simulink model "ThreeDOF_cs"  (Simulink 8.8)
settings: Solver=ode5  StartTime=0.0  StopTime=inf  FixedStep=1/20  RelTol=1e-3
model workspace (MAT data in the model file):
  mbox_table : struct (value not decoded)
  model_closed = 0
  sim_status = 0
PreLoadFcn:
  | check_NUTS_defined;
  | 
  | assignin('base',['model_closed_' bdroot],false);
InitFcn:
  | PreScanExperimentInitFcn(bdroot)
StopFcn:
  | PreScanExperimentStopFcn(bdroot)
undefined symbols (not defined in the file): DiscIntNeverNeededParam, InitImageOutputDir
libraries: PreScanSimulinkLibrary x6, PreScanUsefulBlocks x3
(part 1 of 2)
CloseFcn:
  | evalin('base',['clear model_closed_' bdroot]);
settings Model: Creator=PRESCAN  LastModifiedBy=yuntao891011
settings OptimizationCC: ExpressionDepthLimit=2147483647  InitFltsAndDblsToZero=on
settings DebuggingCC: SaveWithParameterizedLinksMsg=none  SignalResolutionControl=TryResolveAllWithWarning  MultiTaskDSMMsg=warning  MultiTaskCondExecSysMsg=none
settings GRTTargetCC: TargetFcnLib=ansi_tfl_tmw.mat

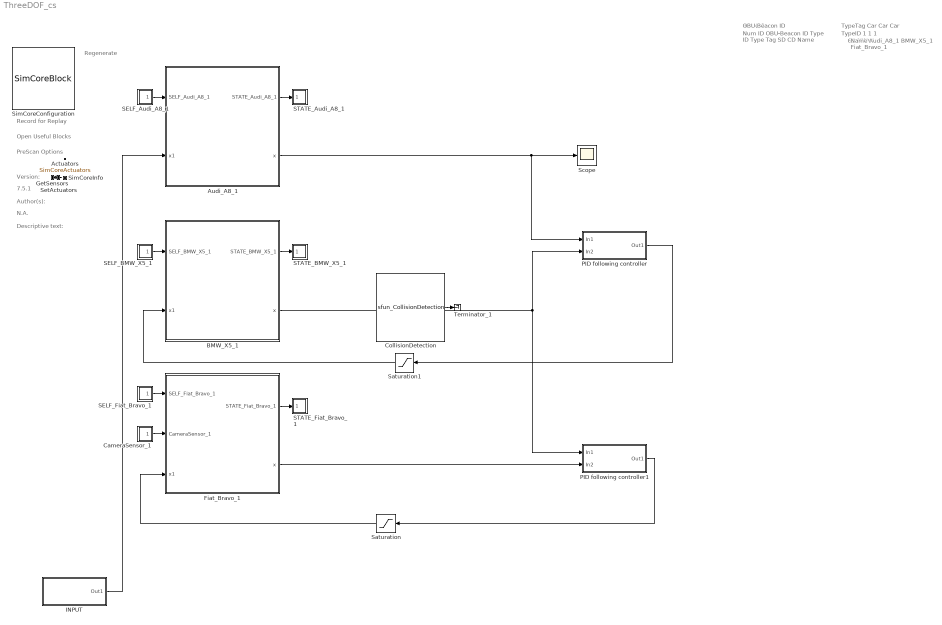
== system ThreeDOF_cs ==
  note: Regenerate
  note: Record for Replay
  note: Open Useful Blocks
  note: PreScan Options
  note: Version:
  note: 7.5.1
  note: Author(s):
  note: N.A.
  note: Descriptive text:
  note: Num ID OBU-Beacon ID Type ID Type Tag SD CD Name
  note: ID
      |
      | 1
      | 2
      | 3
  note: OBU-Beacon ID
  note: TypeID
      |
      | 1
      | 1
      | 1
  note: TypeTag
      |
      | Car
      | Car
      | Car
  note: SD
      |
      | Y
      | Y
      | Y
  note: CD
      |
      | N
      | N
      | N
  note: Name
      |
      | Audi_A8_1
      | BMW_X5_1
      | Fiat_Bravo_1
  Actuators : DataStoreMemory  DataStoreName=SimCoreActuators  InitialValue=zeros(45,1)  ShowAdditionalParam=off
  Audi_A8_1 : Subsystem  Tag=WorldObjectSubSystem  InitFcn=UniqueId = '13';
      mask Display: image(imread('Audi_A8.jpg'));color('white');text(0,0,' ID=1\n')
  BMW_X5_1 : Subsystem  Tag=WorldObjectSubSystem  InitFcn=UniqueId = '14';
      mask Display: image(imread('BMW_X5.jpg'));color('white');text(0,0,' ID=2\n')
  CameraSensor_1 : Subsystem  Tag=CameraSensor  Priority=3  mask(PreScan Source Block: Camera Sensor){}
      mask help: The Camera Sensor provides a color or monochrome image.
      settings: DeleteFcn=PreScanBlockDeleteFcn;
      mask Help: eval('openHelp(457)')
      mask Display: image(imread('CameraSensor.png'))
  CollisionDetection : S-Function  Priority=3  LoadFcn=load('PrescanCollisionDetectionData.mat');load('PrescanCollisionDetectionMessage.mat')  FunctionName=sfun_CollisionDetection  Parameters=timestepMask maxInputMessages maxOutputMessages maxCollisions  SFunctionDeploymentMode=off  EnableBusSupport=off  mask{timestepMask=1/20, maxInputMessages=0, maxOutputMessages=5, maxCollisions=5}
      mask prompts: timestepMask "MATLAB timestep:"; maxInputMessages "Max input messages:"; maxOutputMessages "Max output messages:"; maxCollisions "Maximum number of collisions:"
      mask help: Collision detection output
      mask Display: image(imread('crash.jpg'))
  Fiat_Bravo_1 : Subsystem  Tag=WorldObjectSubSystem  InitFcn=UniqueId = '15';
      mask Display: image(imread('Fiat_Bravo.jpg'));color('white');text(0,0,' ID=3\n')
  GetSensors : Subsystem  Tag=GetSensors  Priority=2  mask(PreScan Simulation Core Block){NrOfSensors=34, TimeStep=1/20}
      mask prompts: NrOfSensors "Number of sensor values"; TimeStep "Timestep [s]"
      mask help:
      | Please do not remove this block from the PreScan compilation sheet,
      | as it contains essential configuration parameters for a PreScan simulation.
      settings: DeleteFcn=PreScanBlockDeleteFcn;
  "INPUT " : Subsystem
  PID following controller : Subsystem
  PID following controller1 : Subsystem
  SELF_Audi_A8_1 : Subsystem  Tag=SELF  Priority=3  mask(PreScan Source Block: SELF){PortName=SELF_Audi_A8_1, PortIndex=10, PortWidth=8, TimeStep=1/20}
      mask prompts: PortName "Auto-Assigned: Port Name [-]"; PortIndex "Auto-Assigned: Port Index [-]"; PortWidth "Auto-Assigned: Port Dimensions"; TimeStep "Auto-Assigned: Upload Period [s]"
      mask help:
      | The SELF port shows (state) information of the actor itself. The outputs are position in the experiment's axis system and the GPS coordinates, and the object's absolute velocity and compass heading.
      |
      | For more information, please click Help.
      settings: DeleteFcn=PreScanBlockDeleteFcn;
      mask Help: eval('openHelp(462)')
      mask Display: image(imread('GPS.png'))
  SELF_BMW_X5_1 : Subsystem  Tag=SELF  Priority=3  mask(PreScan Source Block: SELF){PortName=SELF_BMW_X5_1, PortIndex=18, PortWidth=8, TimeStep=1/20}
      mask prompts: PortName "Auto-Assigned: Port Name [-]"; PortIndex "Auto-Assigned: Port Index [-]"; PortWidth "Auto-Assigned: Port Dimensions"; TimeStep "Auto-Assigned: Upload Period [s]"
      mask help:
      | The SELF port shows (state) information of the actor itself. The outputs are position in the experiment's axis system and the GPS coordinates, and the object's absolute velocity and compass heading.
      |
      | For more information, please click Help.
      settings: DeleteFcn=PreScanBlockDeleteFcn;
      mask Help: eval('openHelp(462)')
      mask Display: image(imread('GPS.png'))
  SELF_Fiat_Bravo_1 : Subsystem  Tag=SELF  Priority=3  mask(PreScan Source Block: SELF){PortName=SELF_Fiat_Bravo_1, PortIndex=26, PortWidth=8, TimeStep=1/20}
      mask prompts: PortName "Auto-Assigned: Port Name [-]"; PortIndex "Auto-Assigned: Port Index [-]"; PortWidth "Auto-Assigned: Port Dimensions"; TimeStep "Auto-Assigned: Upload Period [s]"
      mask help:
      | The SELF port shows (state) information of the actor itself. The outputs are position in the experiment's axis system and the GPS coordinates, and the object's absolute velocity and compass heading.
      |
      | For more information, please click Help.
      settings: DeleteFcn=PreScanBlockDeleteFcn;
      mask Help: eval('openHelp(462)')
      mask Display: image(imread('GPS.png'))
  STATE_Audi_A8_1 : Subsystem  Tag=State  Priority=0  mask(PreScan Sink Block: State){x0=-285.53961181640625, y0=161.16075134277344, z0=0.55, Roll0=0, Pitch0=0, Yaw0=0, TimeStep=1/20}
      mask prompts: x0 "Ini x-position VEHICLE wrt GLOBAL axis system [m]"; y0 "Ini y-position VEHICLE wrt GLOBAL axis system [m]"; z0 "Ini z-position VEHICLE wrt GLOBAL axis system [m]"; Roll0 "Ini roll-angle BODY wrt VEHICLE axis system [deg]"; Pitch0 "Ini pitch-angle BODY wrt VEHICLE axis system [deg]"; Yaw0 "Ini yaw-angle VEHICLE wrt GLOBAL axis system [deg]"; TimeStep "Time Step [s]"
      mask help:
      | The Actor State contains a vector signal of size (9x1), containing the following signals:
      |
      | -  Position                  (x,y,z)                                     [m]
      | -  Velocity                  (vx,vy,vz)                               [m/s]
      | -  Angles                    (Roll, Pitch, Yaw)                   [rad]
      |
      | The Actor state is defined in the global axis system.
      | The state is superponed on the Initial position defined in the GUI.
      |
      | For more information, please click Help.
      settings: DeleteFcn=PreScanBlockDeleteFcn;
      mask Help: eval('openHelp(222)')
      mask Display: image(imread('State.png'))
  STATE_BMW_X5_1 : Subsystem  Tag=State  Priority=0  mask(PreScan Sink Block: State){x0=-302.71296691894531, y0=161.22580718994141, z0=0.69, Roll0=0, Pitch0=0, Yaw0=0, TimeStep=1/20}
      mask prompts: x0 "Ini x-position VEHICLE wrt GLOBAL axis system [m]"; y0 "Ini y-position VEHICLE wrt GLOBAL axis system [m]"; z0 "Ini z-position VEHICLE wrt GLOBAL axis system [m]"; Roll0 "Ini roll-angle BODY wrt VEHICLE axis system [deg]"; Pitch0 "Ini pitch-angle BODY wrt VEHICLE axis system [deg]"; Yaw0 "Ini yaw-angle VEHICLE wrt GLOBAL axis system [deg]"; TimeStep "Time Step [s]"
      mask help:
      | The Actor State contains a vector signal of size (9x1), containing the following signals:
      |
      | -  Position                  (x,y,z)                                     [m]
      | -  Velocity                  (vx,vy,vz)                               [m/s]
      | -  Angles                    (Roll, Pitch, Yaw)                   [rad]
      |
      | The Actor state is defined in the global axis system.
      | The state is superponed on the Initial position defined in the GUI.
      |
      | For more information, please click Help.
      settings: DeleteFcn=PreScanBlockDeleteFcn;
      mask Help: eval('openHelp(222)')
      mask Display: image(imread('State.png'))
  STATE_Fiat_Bravo_1 : Subsystem  Tag=State  Priority=0  mask(PreScan Sink Block: State){x0=-335.43427658081055, y0=161.13351058959961, z0=0.56, Roll0=0, Pitch0=0, Yaw0=0, TimeStep=1/20}
      mask prompts: x0 "Ini x-position VEHICLE wrt GLOBAL axis system [m]"; y0 "Ini y-position VEHICLE wrt GLOBAL axis system [m]"; z0 "Ini z-position VEHICLE wrt GLOBAL axis system [m]"; Roll0 "Ini roll-angle BODY wrt VEHICLE axis system [deg]"; Pitch0 "Ini pitch-angle BODY wrt VEHICLE axis system [deg]"; Yaw0 "Ini yaw-angle VEHICLE wrt GLOBAL axis system [deg]"; TimeStep "Time Step [s]"
      mask help:
      | The Actor State contains a vector signal of size (9x1), containing the following signals:
      |
      | -  Position                  (x,y,z)                                     [m]
      | -  Velocity                  (vx,vy,vz)                               [m/s]
      | -  Angles                    (Roll, Pitch, Yaw)                   [rad]
      |
      | The Actor state is defined in the global axis system.
      | The state is superponed on the Initial position defined in the GUI.
      |
      | For more information, please click Help.
      settings: DeleteFcn=PreScanBlockDeleteFcn;
      mask Help: eval('openHelp(222)')
      mask Display: image(imread('State.png'))
  Saturation : Saturate  UpperLimit=500000  LowerLimit=0
  Saturation1 : Saturate  UpperLimit=500000  LowerLimit=0
  Scope : Scope
  SetActuators : Subsystem  Tag=SetActuators  Priority=1  mask(PreScan Simulation Core Block){TimeStep=1/20, NrOfActuators=45}
      mask prompts: TimeStep "Timestep [s]"; NrOfActuators "Number of actuator values"
      mask help:
      | Please do not remove this block from the PreScan compilation sheet,
      | as it contains essential configuration parameters for a PreScan simulation.
      settings: DeleteFcn=PreScanBlockDeleteFcn;
  SimCoreConfiguration : M-S-Function  Tag=SimCoreConfiguration  Description=DCF5FC37DC6E3E0771C04F3D96D36F9DC5DBC8E5EB9AF2FE837AFFEB0A0E8AE8  FunctionName=SimCoreBlock  Parameters=ExperimentXML PortsXML SimulationCore HostName CheckStart EnableLog RfR EnableGPUAccel ShowComputationTime  mask(PreScan Simulation Core Configurator){SimulationCore=NUTS, HostName=0, CheckStart=0, prescanversion='7.5.1', EnableLog=off, RfR=0, EnableGPUAccel=off, ShowComputationTime=off}
      mask prompts: SimulationCore "Simulation Core"; HostName "Simulation Host"; CheckStart "Show START Dialog"; prescanversion "PreScan Version"; EnableLog "Create TA Log"; RfR "Record for Replay"; EnableGPUAccel "Enable GPU Acceleration"; ShowComputationTime "Show ComputationTime Scope"
      mask help:
      | Please do not remove this block from the PreScan compilation sheet,
      | as it contains essential configuration parameter for a PreScan simulation.
      mask init:
      | model = bdroot;
      | ExperimentXML = [model(1:end-3) '.pex'];
      | PortsXML = [model '_ports.pcd'];
      settings: DeleteFcn=PreScanBlockDeleteFcn;  ModelCloseFcn=assignin('base',['model_closed_' bdroot],true);
      mask Help: eval('openHelp(812)')
      mask Display: image(imread('prescanlogo.ico'))
  SimCoreInfo : Subsystem  Tag=SimCoreInfo
  Terminator_1 : Terminator
  wires:
  SetActuators/1(dummy) -> GetSensors/1(dummy)
  Audi_A8_1/2(x) -> PID following controller/1(In1), Scope/1
  BMW_X5_1/2(x) -> PID following controller1/1(In1), PID following controller/2(In2)
  PID following controller/1(Out1) -> Saturation1/1
  Fiat_Bravo_1/2(x) -> PID following controller1/2(In2)
  PID following controller1/1(Out1) -> Saturation/1
  "INPUT "/1(Out1) -> Audi_A8_1/2(x1)
  Saturation1/1 -> BMW_X5_1/2(x1)
  Saturation/1 -> Fiat_Bravo_1/3(x1)
  Audi_A8_1/1(STATE_Audi_A8_1) -> STATE_Audi_A8_1/1(State)
  SELF_Audi_A8_1/1(U) -> Audi_A8_1/1(SELF_Audi_A8_1)
  BMW_X5_1/1(STATE_BMW_X5_1) -> STATE_BMW_X5_1/1(State)
  SELF_BMW_X5_1/1(U) -> BMW_X5_1/1(SELF_BMW_X5_1)
  Fiat_Bravo_1/1(STATE_Fiat_Bravo_1) -> STATE_Fiat_Bravo_1/1(State)
  SELF_Fiat_Bravo_1/1(U) -> Fiat_Bravo_1/1(SELF_Fiat_Bravo_1)
  CameraSensor_1/1(U1) -> Fiat_Bravo_1/2(CameraSensor_1)
  CollisionDetection/1 -> Terminator_1/1

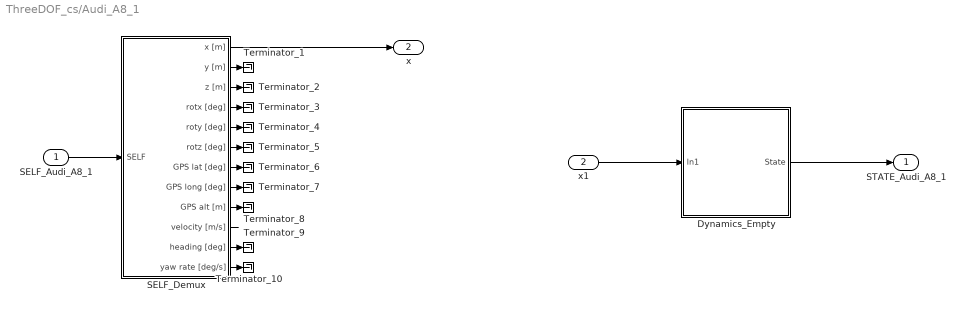
== system ThreeDOF_cs/Audi_A8_1 ==
  SELF_Audi_A8_1 : Inport  Tag=SELFInport
  x1 : Inport  Port=2
  Dynamics_Empty : Subsystem  Tag=Dynamics_Empty
      mask Display: port_label('output', 1, 'State');text(0,0,' Empty\n')
  SELF_Demux : Subsystem  Tag=DemuxSELF  mask(PreScan Demux Block:){}
      settings: DeleteFcn=PreScanBlockDeleteFcn;
      mask Display:
      | port_label('output',1,'x [m]')
      | port_label('output',2,'y [m]')
      | port_label('output',3,'z [m]','texmode','on')
      | port_label('output',4,'Rotx [deg]','texmode','on')
      | port_label('output',5,'Roty [deg]','texmode','on')
      | port_label('output',6,'Rotz [deg]','texmode','on')
      | port_label('output',7,'GPS lat [deg]','texmode','on')
      | port_label('output',8,'GPS long [deg]','texmode','on')
      | port_label('output',9,'GPS alt [m]','texmode','on')
      | port_label('output',10,'Velocity [m/s]')
      | port_label('output',11,'Heading [deg]')
      | port_label('output',12,'Yaw rate [deg/s]')
  Terminator_{1..10} (10 alike) : Terminator
  STATE_Audi_A8_1 : Outport  Tag=StateOutport
  x : Outport  Port=2
  wires:
  SELF_Demux/1(x [m]) -> x/1
  SELF_Demux/10(velocity [m/s]) -> ?
  x1/1 -> Dynamics_Empty/1(In1)
  SELF_Audi_A8_1/1 -> SELF_Demux/1(SELF)
  Dynamics_Empty/1(State) -> STATE_Audi_A8_1/1
  SELF_Demux/2(y [m]) -> Terminator_1/1
  SELF_Demux/3(z [m]) -> Terminator_2/1
  SELF_Demux/4(rotx [deg]) -> Terminator_3/1
  SELF_Demux/5(roty [deg]) -> Terminator_4/1
  SELF_Demux/6(rotz [deg]) -> Terminator_5/1
  SELF_Demux/7(GPS lat [deg]) -> Terminator_6/1
  SELF_Demux/8(GPS long [deg]) -> Terminator_7/1
  SELF_Demux/9(GPS alt [m]) -> Terminator_8/1
  SELF_Demux/11(heading [deg]) -> Terminator_9/1
  SELF_Demux/12(yaw rate [deg/s]) -> Terminator_10/1

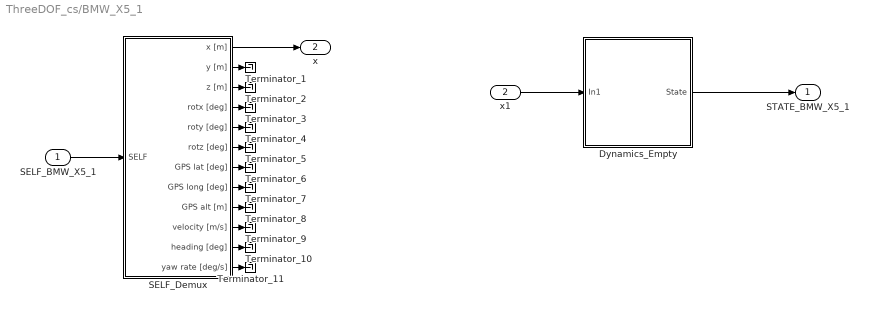
== system ThreeDOF_cs/BMW_X5_1 ==
  SELF_BMW_X5_1 : Inport  Tag=SELFInport
  x1 : Inport  Port=2
  Dynamics_Empty : Subsystem  Tag=Dynamics_Empty
      mask Display: port_label('output', 1, 'State');text(0,0,' Empty\n')
  SELF_Demux : Subsystem  Tag=DemuxSELF  mask(PreScan Demux Block:){}
      settings: DeleteFcn=PreScanBlockDeleteFcn;
      mask Display:
      | port_label('output',1,'x [m]')
      | port_label('output',2,'y [m]')
      | port_label('output',3,'z [m]','texmode','on')
      | port_label('output',4,'Rotx [deg]','texmode','on')
      | port_label('output',5,'Roty [deg]','texmode','on')
      | port_label('output',6,'Rotz [deg]','texmode','on')
      | port_label('output',7,'GPS lat [deg]','texmode','on')
      | port_label('output',8,'GPS long [deg]','texmode','on')
      | port_label('output',9,'GPS alt [m]','texmode','on')
      | port_label('output',10,'Velocity [m/s]')
      | port_label('output',11,'Heading [deg]')
      | port_label('output',12,'Yaw rate [deg/s]')
  Terminator_{1..11} (11 alike) : Terminator
  STATE_BMW_X5_1 : Outport  Tag=StateOutport
  x : Outport  Port=2
  wires:
  SELF_Demux/1(x [m]) -> x/1
  x1/1 -> Dynamics_Empty/1(In1)
  SELF_BMW_X5_1/1 -> SELF_Demux/1(SELF)
  Dynamics_Empty/1(State) -> STATE_BMW_X5_1/1
  SELF_Demux/2(y [m]) -> Terminator_1/1
  SELF_Demux/3(z [m]) -> Terminator_2/1
  SELF_Demux/4(rotx [deg]) -> Terminator_3/1
  SELF_Demux/5(roty [deg]) -> Terminator_4/1
  SELF_Demux/6(rotz [deg]) -> Terminator_5/1
  SELF_Demux/7(GPS lat [deg]) -> Terminator_6/1
  SELF_Demux/8(GPS long [deg]) -> Terminator_7/1
  SELF_Demux/9(GPS alt [m]) -> Terminator_8/1
  SELF_Demux/10(velocity [m/s]) -> Terminator_9/1
  SELF_Demux/11(heading [deg]) -> Terminator_10/1
  SELF_Demux/12(yaw rate [deg/s]) -> Terminator_11/1

== system ThreeDOF_cs/CameraSensor_1 ==
  Demux : Demux  Outputs=[1 -1]
  Terminator : Terminator
  U1 : Outport
  wires:
  Demux/2 -> Terminator/1
  Demux/1 -> U1/1
  [SimCoreSensors] -> Demux/1

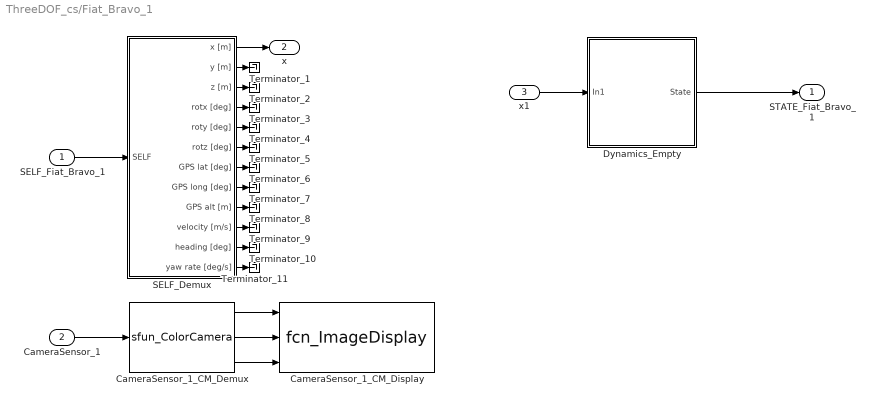
== system ThreeDOF_cs/Fiat_Bravo_1 ==
  SELF_Fiat_Bravo_1 : Inport  Tag=SELFInport
  CameraSensor_1 : Inport  Tag=CameraSensorInport  Port=2  SampleTime=1/20
  x1 : Inport  Port=3
  CameraSensor_1_CM_Demux : S-Function  Tag=CameraSensor_Color_Demux  FunctionName=sfun_ColorCamera  Parameters=[VerticalResolution HorizontalResolution] FrameRate SensorName CameraType SharedMemTag SharedMemRightTag DataType  SFunctionDeploymentMode=off  EnableBusSupport=off  mask{HorizontalResolution=500, VerticalResolution=375, FrameRate=20, SensorName=CameraSensor_1, CameraType=Mono, SharedMemTag=CameraSensor_1_monoBeam_viewer_RGB, SharedMemRightTag=CameraSensor_1_StereoRight_viewer_RGB, DataType=uint8}
      mask prompts: HorizontalResolution "User Specified: Horizontal Resolution [pixels]"; VerticalResolution "User Specified: Vertical Resolution [pixels]"; FrameRate "User Specified: Frame Rate [Hz]"; SensorName "User Specified: Camera Sensor Name"; CameraType "Camera Type"; SharedMemTag "Tag for shared memory for main img"; SharedMemRightTag "Tag for shared memory for right img"; DataType "Image Data Type"
      mask init:
      | if CameraType==1
      |     CameraTypeName='MONO';
      |     PortNumber=0;
      | else
      |     CameraTypeName='STEREO';
      |     PortNumber=3;
      | end
      settings: DeleteFcn=PreScanBlockDeleteFcn;
      mask TypeOptions CameraType: Mono | Stereo
      mask TypeOptions DataType: uint8 | single
      mask Display:
      | fprintf('%s CAMERA:\n Color\n %s \n V: %d x %d \n %d fps',CameraTypeName,SensorName,VerticalResolution,HorizontalResolution,FrameRate)
      | port_label('output',1,'R')
      | port_label('output',2,'G')
      | port_label('output',3,'B')
      | port_label('output',PortNumber+1,'R')
      | port_label('output',PortNumber+2,'G')
      | port_label('output',PortNumber+3,'B')
  CameraSensor_1_CM_Display : M-S-Function  Tag=CameraSensor_Color_Display  InitFcn=InitImageOutputDir(gcb);  FunctionName=fcn_ImageDisplay  Parameters=SensorName EnableDisplay EnablePosition DisplayPosition FigureHandle SaveResults BitmapFormat TempOutputDir CameraType DataType  mask(PreScan Color Display Block){SensorName=CameraSensor_1, EnableDisplay=on, EnablePosition=off, DisplayPosition=[10 10 500 375], FigureHandle=300, SaveResults=off, Format=PNG, TempOutputDir=0, CameraType=Mono, DataType=uint8}
      mask prompts: SensorName "User Specified: Title of Display"; EnableDisplay "Active"; EnablePosition "Set Display window position"; DisplayPosition "Display window position [xpos ypos width height]"; FigureHandle "Unique Handle"; SaveResults "Save results"; TempOutputDir "OutputDir"; CameraType "Camera Type"; DataType "Image Data Type"
      mask help: This block displays the RGB output of a PreScan camera sensor.
      mask init:
      | if EnableDisplay
      |     EnableString='';
      |     EnableColor='gray';
      | else
      |     EnableString='INACTIVE';
      |     EnableColor='red';
      | end
      | switch Format
      |     case 1
      |         BitmapFormat = 'png';
      |     case 2
      |         BitmapFormat = 'bmp';
      |     case 3
      |         BitmapFormat = 'jpg';
      | end 
      | if CameraType==1
      |     CameraTypeName='MONO';
      |     PortNumber=0;
      | else
      |     CameraTypeName='STEREO';
      |     PortNumber=3;
      | end
      settings: CopyFcn=CopyFcnDisplay  DeleteFcn=PreScanBlockDeleteFcn;  ModelCloseFcn=fcn_ImageDisplay_ModelCloseFcn
      mask Help: eval('openHelp(457)')
      mask Callback EnablePosition:
      | MV=get_param(gcb,'MaskVisibilities');
      | if strcmp(get_param(gcb,'EnablePosition'),'on')
      |     MV{4}='on';
      | else
      |     MV{4}='off';
      | end
      | set_param(gcb,'MaskVisibilities',MV);
      mask TypeOptions Format: PNG | BMP | JPG
      mask TypeOptions CameraType: Mono | Stereo
      mask TypeOptions DataType: uint8 | single
      mask Display:
      | color(EnableColor);
      | fprintf('%s\n DISPLAY:\n Color \n %s',EnableString,SensorName)
      | port_label('input',1,'R')
      | port_label('input',2,'G')
      | port_label('input',3,'B')
      | port_label('input',PortNumber+1,'R')
      | port_label('input',PortNumber+2,'G')
      | port_label('input',PortNumber+3,'B')
  Dynamics_Empty : Subsystem  Tag=Dynamics_Empty
      mask Display: port_label('output', 1, 'State');text(0,0,' Empty\n')
  SELF_Demux : Subsystem  Tag=DemuxSELF  mask(PreScan Demux Block:){}
      settings: DeleteFcn=PreScanBlockDeleteFcn;
      mask Display:
      | port_label('output',1,'x [m]')
      | port_label('output',2,'y [m]')
      | port_label('output',3,'z [m]','texmode','on')
      | port_label('output',4,'Rotx [deg]','texmode','on')
      | port_label('output',5,'Roty [deg]','texmode','on')
      | port_label('output',6,'Rotz [deg]','texmode','on')
      | port_label('output',7,'GPS lat [deg]','texmode','on')
      | port_label('output',8,'GPS long [deg]','texmode','on')
      | port_label('output',9,'GPS alt [m]','texmode','on')
      | port_label('output',10,'Velocity [m/s]')
      | port_label('output',11,'Heading [deg]')
      | port_label('output',12,'Yaw rate [deg/s]')
  Terminator_{1..11} (11 alike) : Terminator
  STATE_Fiat_Bravo_1 : Outport  Tag=StateOutport
  x : Outport  Port=2
  wires:
  SELF_Demux/1(x [m]) -> x/1
  x1/1 -> Dynamics_Empty/1(In1)
  SELF_Fiat_Bravo_1/1 -> SELF_Demux/1(SELF)
  CameraSensor_1_CM_Demux/1 -> CameraSensor_1_CM_Display/1
  CameraSensor_1_CM_Demux/2 -> CameraSensor_1_CM_Display/2
  CameraSensor_1_CM_Demux/3 -> CameraSensor_1_CM_Display/3
  CameraSensor_1/1 -> CameraSensor_1_CM_Demux/1
  Dynamics_Empty/1(State) -> STATE_Fiat_Bravo_1/1
  SELF_Demux/2(y [m]) -> Terminator_1/1
  SELF_Demux/3(z [m]) -> Terminator_2/1
  SELF_Demux/4(rotx [deg]) -> Terminator_3/1
  SELF_Demux/5(roty [deg]) -> Terminator_4/1
  SELF_Demux/6(rotz [deg]) -> Terminator_5/1
  SELF_Demux/7(GPS lat [deg]) -> Terminator_6/1
  SELF_Demux/8(GPS long [deg]) -> Terminator_7/1
  SELF_Demux/9(GPS alt [m]) -> Terminator_8/1
  SELF_Demux/10(velocity [m/s]) -> Terminator_9/1
  SELF_Demux/11(heading [deg]) -> Terminator_10/1
  SELF_Demux/12(yaw rate [deg/s]) -> Terminator_11/1

== system ThreeDOF_cs/GetSensors ==
  dummy : Inport
  GetSensors : M-S-Function  FunctionName=GetSensorsBlock  Parameters=TimeStep NrOfSensors
  tag scope: SimCoreSensors=global
  wires:
  GetSensors/1 -> [SimCoreSensors]
  dummy/1 -> GetSensors/1

== system ThreeDOF_cs/INPUT  ==
  Scope : Scope
  Sine Wave : Sin  Amplitude=2  Bias=2.5  Frequency=0.4  SampleTime=0
  Out1 : Outport
  wires:
  Sine Wave/1 -> Scope/1, Out1/1

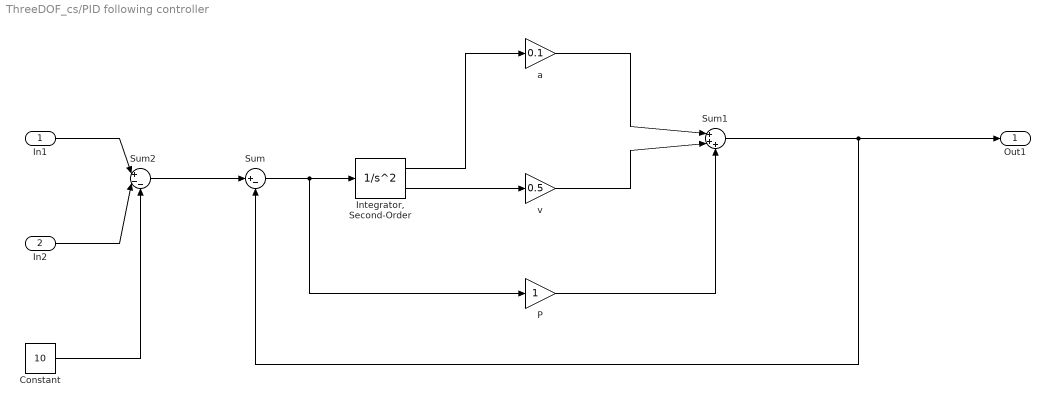
== system ThreeDOF_cs/PID following controller ==
  In1 : Inport
  In2 : Inport  Port=2
  Constant : Constant  Value=10
  "Integrator, Second-Order" : SecondOrderIntegrator
  P : Gain
  Sum : Sum  Inputs=|+-
  Sum1 : Sum  Inputs=|+++
  Sum2 : Sum  Inputs=|+--
  a : Gain  Gain=0.1
  v : Gain  Gain=0.5
  Out1 : Outport
  wires:
  Sum/1 -> P/1, "Integrator, Second-Order"/1
  "Integrator, Second-Order"/1 -> a/1
  "Integrator, Second-Order"/2 -> v/1
  a/1 -> Sum1/1
  v/1 -> Sum1/2
  P/1 -> Sum1/3
  Sum1/1 -> Out1/1, Sum/2
  In1/1 -> Sum2/1
  Sum2/1 -> Sum/1
  In2/1 -> Sum2/2
  Constant/1 -> Sum2/3

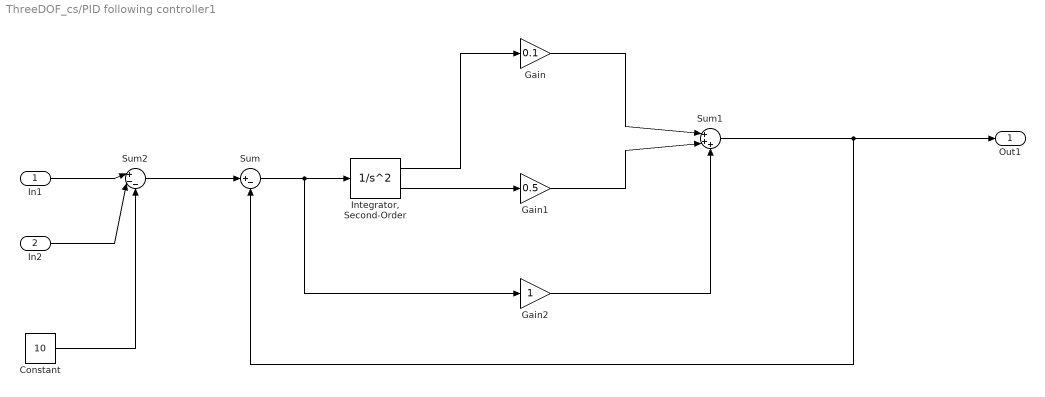
== system ThreeDOF_cs/PID following controller1 ==
  In1 : Inport
  In2 : Inport  Port=2
  Constant : Constant  Value=10
  Gain : Gain  Gain=0.1
  Gain1 : Gain  Gain=0.5
  Gain2 : Gain
  "Integrator, Second-Order" : SecondOrderIntegrator
  Sum : Sum  Inputs=|+-
  Sum1 : Sum  Inputs=|+++
  Sum2 : Sum  Inputs=|+--
  Out1 : Outport
  wires:
  Sum/1 -> Gain2/1, "Integrator, Second-Order"/1
  "Integrator, Second-Order"/1 -> Gain/1
  "Integrator, Second-Order"/2 -> Gain1/1
  Gain/1 -> Sum1/1
  Gain1/1 -> Sum1/2
  Gain2/1 -> Sum1/3
  Sum1/1 -> Out1/1, Sum/2
  In1/1 -> Sum2/1
  Sum2/1 -> Sum/1
  In2/1 -> Sum2/2
  Constant/1 -> Sum2/3

== system ThreeDOF_cs/SELF_Audi_A8_1 ==
  Selector : Selector  IndexMode=Zero-based  IndexOptions=Starting index (dialog)  Indices=PortIndex  OutputSizes=PortWidth(1)
  U : Outport
  wires:
  Selector/1 -> U/1
  [SimCoreSensors] -> Selector/1

== system ThreeDOF_cs/SELF_BMW_X5_1 ==
  Selector : Selector  IndexMode=Zero-based  IndexOptions=Starting index (dialog)  Indices=PortIndex  OutputSizes=PortWidth(1)
  U : Outport
  wires:
  Selector/1 -> U/1
  [SimCoreSensors] -> Selector/1

== system ThreeDOF_cs/SELF_Fiat_Bravo_1 ==
  Selector : Selector  IndexMode=Zero-based  IndexOptions=Starting index (dialog)  Indices=PortIndex  OutputSizes=PortWidth(1)
  U : Outport
  wires:
  Selector/1 -> U/1
  [SimCoreSensors] -> Selector/1

== system ThreeDOF_cs/STATE_Audi_A8_1 ==
  State : Inport  SampleTime=TimeStep
  Acceleration : Subsystem  mask(ToSensorWorld){PortName=Acceleration_Audi_A8_1, PortIndex=6, PortWidth=3, TimeStep=1/20}
      mask prompts: PortName "Port Name [-]"; PortIndex "Index [-]"; PortWidth "Port Dimensions [-]"; TimeStep "Upload Period [s]"
      mask help: Sends signal(s) from Simulink to the Sensor World
      mask Help:
      | Sends signal(s) from Simulink to the Sensor World.
      | 
      | - Port Name [-]: specifies the name of the output terminal of the Simulink block.
      | - Index [-]: specifies the start position in the output vector sent to the Sensor World
      | - Port dimensions [-]: specifies the width (number of scalars) of the output port
      | - Upload period [s]: specifies the upload period (in seconds) of the port.
      mask Display: port_label('input', 1, PortName)
  Demux : Demux  Outputs=5
  Position : Subsystem  mask(ToSensorWorld){PortName=Position_Audi_A8_1, PortIndex=0, PortWidth=3, TimeStep=1/20}
      mask prompts: PortName "Port Name [-]"; PortIndex "Index [-]"; PortWidth "Port Dimensions [-]"; TimeStep "Upload Period [s]"
      mask help: Sends signal(s) from Simulink to the Sensor World
      mask Help:
      | Sends signal(s) from Simulink to the Sensor World.
      | 
      | - Port Name [-]: specifies the name of the output terminal of the Simulink block.
      | - Index [-]: specifies the start position in the output vector sent to the Sensor World
      | - Port dimensions [-]: specifies the width (number of scalars) of the output port
      | - Upload period [s]: specifies the upload period (in seconds) of the port.
      mask Display: port_label('input', 1, PortName)
  RPY : Subsystem  mask(ToSensorWorld){PortName=RPY_Audi_A8_1, PortIndex=9, PortWidth=3, TimeStep=1/20}
      mask prompts: PortName "Port Name [-]"; PortIndex "Index [-]"; PortWidth "Port Dimensions [-]"; TimeStep "Upload Period [s]"
      mask help: Sends signal(s) from Simulink to the Sensor World
      mask Help:
      | Sends signal(s) from Simulink to the Sensor World.
      | 
      | - Port Name [-]: specifies the name of the output terminal of the Simulink block.
      | - Index [-]: specifies the start position in the output vector sent to the Sensor World
      | - Port dimensions [-]: specifies the width (number of scalars) of the output port
      | - Upload period [s]: specifies the upload period (in seconds) of the port.
      mask Display: port_label('input', 1, PortName)
  Velocity : Subsystem  mask(ToSensorWorld){PortName=Velocity_Audi_A8_1, PortIndex=3, PortWidth=3, TimeStep=1/20}
      mask prompts: PortName "Port Name [-]"; PortIndex "Index [-]"; PortWidth "Port Dimensions [-]"; TimeStep "Upload Period [s]"
      mask help: Sends signal(s) from Simulink to the Sensor World
      mask Help:
      | Sends signal(s) from Simulink to the Sensor World.
      | 
      | - Port Name [-]: specifies the name of the output terminal of the Simulink block.
      | - Index [-]: specifies the start position in the output vector sent to the Sensor World
      | - Port dimensions [-]: specifies the width (number of scalars) of the output port
      | - Upload period [s]: specifies the upload period (in seconds) of the port.
      mask Display: port_label('input', 1, PortName)
  iniBODYAngles wrtVEH [rad] : Constant  Value=[Roll0 Pitch0 0]  SampleTime=TimeStep
  iniVEHAngles wrtGLOB [rad] : Constant  Value=[0 0 Yaw0]  SampleTime=TimeStep
  iniVEHposition wrtGLOB [m] : Constant  Value=[x0 y0 z0]  SampleTime=TimeStep
  state2FullState : PreScanSimulinkLibrary/state2FullState  SystemSampleTime=-1
  velRPY : Subsystem  mask(ToSensorWorld){PortName=velRPY_Audi_A8_1, PortIndex=12, PortWidth=3, TimeStep=1/20}
      mask prompts: PortName "Port Name [-]"; PortIndex "Index [-]"; PortWidth "Port Dimensions [-]"; TimeStep "Upload Period [s]"
      mask help: Sends signal(s) from Simulink to the Sensor World
      mask Help:
      | Sends signal(s) from Simulink to the Sensor World.
      | 
      | - Port Name [-]: specifies the name of the output terminal of the Simulink block.
      | - Index [-]: specifies the start position in the output vector sent to the Sensor World
      | - Port dimensions [-]: specifies the width (number of scalars) of the output port
      | - Upload period [s]: specifies the upload period (in seconds) of the port.
      mask Display: port_label('input', 1, PortName)
  wires:
  Demux/5 -> velRPY/1(Y)
  Demux/4 -> RPY/1(Y)
  Demux/3 -> Acceleration/1(Y)
  Demux/2 -> Velocity/1(Y)
  Demux/1 -> Position/1(Y)
  State/1 -> state2FullState/1
  state2FullState/1 -> Demux/1
  iniVEHposition wrtGLOB [m]/1 -> state2FullState/2
  iniBODYAngles wrtVEH [rad]/1 -> state2FullState/3
  iniVEHAngles wrtGLOB [rad]/1 -> state2FullState/4

== system ThreeDOF_cs/STATE_BMW_X5_1 ==
  State : Inport  SampleTime=TimeStep
  Acceleration : Subsystem  mask(ToSensorWorld){PortName=Acceleration_BMW_X5_1, PortIndex=21, PortWidth=3, TimeStep=1/20}
      mask prompts: PortName "Port Name [-]"; PortIndex "Index [-]"; PortWidth "Port Dimensions [-]"; TimeStep "Upload Period [s]"
      mask help: Sends signal(s) from Simulink to the Sensor World
      mask Help:
      | Sends signal(s) from Simulink to the Sensor World.
      | 
      | - Port Name [-]: specifies the name of the output terminal of the Simulink block.
      | - Index [-]: specifies the start position in the output vector sent to the Sensor World
      | - Port dimensions [-]: specifies the width (number of scalars) of the output port
      | - Upload period [s]: specifies the upload period (in seconds) of the port.
      mask Display: port_label('input', 1, PortName)
  Demux : Demux  Outputs=5
  Position : Subsystem  mask(ToSensorWorld){PortName=Position_BMW_X5_1, PortIndex=15, PortWidth=3, TimeStep=1/20}
      mask prompts: PortName "Port Name [-]"; PortIndex "Index [-]"; PortWidth "Port Dimensions [-]"; TimeStep "Upload Period [s]"
      mask help: Sends signal(s) from Simulink to the Sensor World
      mask Help:
      | Sends signal(s) from Simulink to the Sensor World.
      | 
      | - Port Name [-]: specifies the name of the output terminal of the Simulink block.
      | - Index [-]: specifies the start position in the output vector sent to the Sensor World
      | - Port dimensions [-]: specifies the width (number of scalars) of the output port
      | - Upload period [s]: specifies the upload period (in seconds) of the port.
      mask Display: port_label('input', 1, PortName)
  RPY : Subsystem  mask(ToSensorWorld){PortName=RPY_BMW_X5_1, PortIndex=24, PortWidth=3, TimeStep=1/20}
      mask prompts: PortName "Port Name [-]"; PortIndex "Index [-]"; PortWidth "Port Dimensions [-]"; TimeStep "Upload Period [s]"
      mask help: Sends signal(s) from Simulink to the Sensor World
      mask Help:
      | Sends signal(s) from Simulink to the Sensor World.
      | 
      | - Port Name [-]: specifies the name of the output terminal of the Simulink block.
      | - Index [-]: specifies the start position in the output vector sent to the Sensor World
      | - Port dimensions [-]: specifies the width (number of scalars) of the output port
      | - Upload period [s]: specifies the upload period (in seconds) of the port.
      mask Display: port_label('input', 1, PortName)
  Velocity : Subsystem  mask(ToSensorWorld){PortName=Velocity_BMW_X5_1, PortIndex=18, PortWidth=3, TimeStep=1/20}
      mask prompts: PortName "Port Name [-]"; PortIndex "Index [-]"; PortWidth "Port Dimensions [-]"; TimeStep "Upload Period [s]"
      mask help: Sends signal(s) from Simulink to the Sensor World
      mask Help:
      | Sends signal(s) from Simulink to the Sensor World.
      | 
      | - Port Name [-]: specifies the name of the output terminal of the Simulink block.
      | - Index [-]: specifies the start position in the output vector sent to the Sensor World
      | - Port dimensions [-]: specifies the width (number of scalars) of the output port
      | - Upload period [s]: specifies the upload period (in seconds) of the port.
      mask Display: port_label('input', 1, PortName)
  iniBODYAngles wrtVEH [rad] : Constant  Value=[Roll0 Pitch0 0]  SampleTime=TimeStep
  iniVEHAngles wrtGLOB [rad] : Constant  Value=[0 0 Yaw0]  SampleTime=TimeStep
  iniVEHposition wrtGLOB [m] : Constant  Value=[x0 y0 z0]  SampleTime=TimeStep
  state2FullState : PreScanSimulinkLibrary/state2FullState  SystemSampleTime=-1
  velRPY : Subsystem  mask(ToSensorWorld){PortName=velRPY_BMW_X5_1, PortIndex=27, PortWidth=3, TimeStep=1/20}
      mask prompts: PortName "Port Name [-]"; PortIndex "Index [-]"; PortWidth "Port Dimensions [-]"; TimeStep "Upload Period [s]"
      mask help: Sends signal(s) from Simulink to the Sensor World
      mask Help:
      | Sends signal(s) from Simulink to the Sensor World.
      | 
      | - Port Name [-]: specifies the name of the output terminal of the Simulink block.
      | - Index [-]: specifies the start position in the output vector sent to the Sensor World
      | - Port dimensions [-]: specifies the width (number of scalars) of the output port
      | - Upload period [s]: specifies the upload period (in seconds) of the port.
      mask Display: port_label('input', 1, PortName)
  wires:
  Demux/5 -> velRPY/1(Y)
  Demux/4 -> RPY/1(Y)
  Demux/3 -> Acceleration/1(Y)
  Demux/2 -> Velocity/1(Y)
  Demux/1 -> Position/1(Y)
  State/1 -> state2FullState/1
  state2FullState/1 -> Demux/1
  iniVEHposition wrtGLOB [m]/1 -> state2FullState/2
  iniBODYAngles wrtVEH [rad]/1 -> state2FullState/3
  iniVEHAngles wrtGLOB [rad]/1 -> state2FullState/4

== system ThreeDOF_cs/STATE_Fiat_Bravo_1 ==
  State : Inport  SampleTime=TimeStep
  Acceleration : Subsystem  mask(ToSensorWorld){PortName=Acceleration_Fiat_Bravo_1, PortIndex=36, PortWidth=3, TimeStep=1/20}
      mask prompts: PortName "Port Name [-]"; PortIndex "Index [-]"; PortWidth "Port Dimensions [-]"; TimeStep "Upload Period [s]"
      mask help: Sends signal(s) from Simulink to the Sensor World
      mask Help:
      | Sends signal(s) from Simulink to the Sensor World.
      | 
      | - Port Name [-]: specifies the name of the output terminal of the Simulink block.
      | - Index [-]: specifies the start position in the output vector sent to the Sensor World
      | - Port dimensions [-]: specifies the width (number of scalars) of the output port
      | - Upload period [s]: specifies the upload period (in seconds) of the port.
      mask Display: port_label('input', 1, PortName)
  Demux : Demux  Outputs=5
  Position : Subsystem  mask(ToSensorWorld){PortName=Position_Fiat_Bravo_1, PortIndex=30, PortWidth=3, TimeStep=1/20}
      mask prompts: PortName "Port Name [-]"; PortIndex "Index [-]"; PortWidth "Port Dimensions [-]"; TimeStep "Upload Period [s]"
      mask help: Sends signal(s) from Simulink to the Sensor World
      mask Help:
      | Sends signal(s) from Simulink to the Sensor World.
      | 
      | - Port Name [-]: specifies the name of the output terminal of the Simulink block.
      | - Index [-]: specifies the start position in the output vector sent to the Sensor World
      | - Port dimensions [-]: specifies the width (number of scalars) of the output port
      | - Upload period [s]: specifies the upload period (in seconds) of the port.
      mask Display: port_label('input', 1, PortName)
  RPY : Subsystem  mask(ToSensorWorld){PortName=RPY_Fiat_Bravo_1, PortIndex=39, PortWidth=3, TimeStep=1/20}
      mask prompts: PortName "Port Name [-]"; PortIndex "Index [-]"; PortWidth "Port Dimensions [-]"; TimeStep "Upload Period [s]"
      mask help: Sends signal(s) from Simulink to the Sensor World
      mask Help:
      | Sends signal(s) from Simulink to the Sensor World.
      | 
      | - Port Name [-]: specifies the name of the output terminal of the Simulink block.
      | - Index [-]: specifies the start position in the output vector sent to the Sensor World
      | - Port dimensions [-]: specifies the width (number of scalars) of the output port
      | - Upload period [s]: specifies the upload period (in seconds) of the port.
      mask Display: port_label('input', 1, PortName)
  Velocity : Subsystem  mask(ToSensorWorld){PortName=Velocity_Fiat_Bravo_1, PortIndex=33, PortWidth=3, TimeStep=1/20}
      mask prompts: PortName "Port Name [-]"; PortIndex "Index [-]"; PortWidth "Port Dimensions [-]"; TimeStep "Upload Period [s]"
      mask help: Sends signal(s) from Simulink to the Sensor World
      mask Help:
      | Sends signal(s) from Simulink to the Sensor World.
      | 
      | - Port Name [-]: specifies the name of the output terminal of the Simulink block.
      | - Index [-]: specifies the start position in the output vector sent to the Sensor World
      | - Port dimensions [-]: specifies the width (number of scalars) of the output port
      | - Upload period [s]: specifies the upload period (in seconds) of the port.
      mask Display: port_label('input', 1, PortName)
  iniBODYAngles wrtVEH [rad] : Constant  Value=[Roll0 Pitch0 0]  SampleTime=TimeStep
  iniVEHAngles wrtGLOB [rad] : Constant  Value=[0 0 Yaw0]  SampleTime=TimeStep
  iniVEHposition wrtGLOB [m] : Constant  Value=[x0 y0 z0]  SampleTime=TimeStep
  state2FullState : PreScanSimulinkLibrary/state2FullState  SystemSampleTime=-1
  velRPY : Subsystem  mask(ToSensorWorld){PortName=velRPY_Fiat_Bravo_1, PortIndex=42, PortWidth=3, TimeStep=1/20}
      mask prompts: PortName "Port Name [-]"; PortIndex "Index [-]"; PortWidth "Port Dimensions [-]"; TimeStep "Upload Period [s]"
      mask help: Sends signal(s) from Simulink to the Sensor World
      mask Help:
      | Sends signal(s) from Simulink to the Sensor World.
      | 
      | - Port Name [-]: specifies the name of the output terminal of the Simulink block.
      | - Index [-]: specifies the start position in the output vector sent to the Sensor World
      | - Port dimensions [-]: specifies the width (number of scalars) of the output port
      | - Upload period [s]: specifies the upload period (in seconds) of the port.
      mask Display: port_label('input', 1, PortName)
  wires:
  Demux/5 -> velRPY/1(Y)
  Demux/4 -> RPY/1(Y)
  Demux/3 -> Acceleration/1(Y)
  Demux/2 -> Velocity/1(Y)
  Demux/1 -> Position/1(Y)
  State/1 -> state2FullState/1
  state2FullState/1 -> Demux/1
  iniVEHposition wrtGLOB [m]/1 -> state2FullState/2
  iniBODYAngles wrtVEH [rad]/1 -> state2FullState/3
  iniVEHAngles wrtGLOB [rad]/1 -> state2FullState/4

== system ThreeDOF_cs/SetActuators ==
  Bus Creator : BusCreator  Inputs=1
  Data Store Read : DataStoreRead  DataStoreName=SimCoreActuators  SampleTime=TimeStep
  SendActuators : M-S-Function  FunctionName=SendActuatorsBlock  Parameters=TimeStep NrOfActuators
  dummy : Outport
  tag scope: SimCoreInfo=global
  wires:
  Bus Creator/1 -> [SimCoreInfo]  "SimCore"
  SendActuators/2 -> Bus Creator/1  "ComputationTime[s]"
  SendActuators/1 -> dummy/1
  Data Store Read/1 -> SendActuators/1

== system ThreeDOF_cs/SimCoreInfo ==
  Bus Selector : BusSelector  OutputSignals=ComputationTime[s]
  Time : Scope
  wires:
  Bus Selector/1 -> Time/1  "<ComputationTime[s]>"
  [SimCoreInfo] -> Bus Selector/1

== system ThreeDOF_cs/Audi_A8_1/Dynamics_Empty ==
  note: For state mode 'Dynamic' positions
      | are not taken into account, as they
      | are computed by integrating velocity.
      | Click annotation for Help.
  In1 : Inport
  Ground_{1..7} (7 alike) : Ground
  Integrator : Integrator
  MuxState : Subsystem  Tag=MuxState  mask(Empty Dynamics State Block){positioningmode=on, TimeStep=1/20}
      mask prompts: positioningmode "Positioning Mode"; TimeStep "Auto Assigned: Time Step [s]"
      mask help:
      | Build the state of an actor based on user input.
      | The user can either use positioning mode or dynamics mode.
      | - When using positioning mode the position and orientation of the actor are set directly based on the input. Expected input is relative to the initial position and orientation of the actor. It's also possible to specify the velocity of the actor, though this input isn't used, only passed on.
      | - When using dynamics mode the position input is ignored. Expected input is velocity and orientation. The velocity is relative the current orientation of the actor, while orientation is relative to its initial orientation. The position of the actor is calculated based on the velocity and orientation given.
      settings: DeleteFcn=PreScanBlockDeleteFcn;
  State : Outport  Tag=StateOutport
  wires:
  Integrator/1 -> MuxState/1(x [m])
  In1/1 -> Integrator/1, MuxState/4(dx [m/s])
  MuxState/1(state) -> State/1
  Ground_1/1 -> MuxState/2(y [m])
  Ground_2/1 -> MuxState/3(z [m])
  Ground_3/1 -> MuxState/5(dy [m/s])
  Ground_4/1 -> MuxState/6(dz [m/s])
  Ground_5/1 -> MuxState/7(R [rad])
  Ground_6/1 -> MuxState/8(P [rad])
  Ground_7/1 -> MuxState/9(Y [rad])

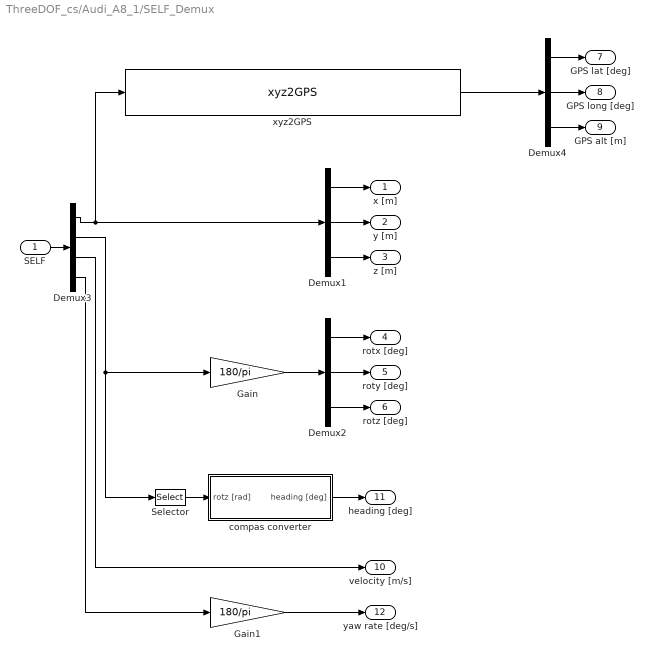
== system ThreeDOF_cs/Audi_A8_1/SELF_Demux ==
  SELF : Inport
  Demux1 : Demux  Outputs=3
  Demux2 : Demux  Outputs=3
  Demux3 : Demux  Outputs=[3 3 1 1]
  Demux4 : Demux  Outputs=3
  Gain : Gain  Gain=180/pi
  Gain1 : Gain  Gain=180/pi
  Selector : Selector  InputPortWidth=3  IndexOptions=Index vector (dialog)  Indices=[3]  OutputSizes=1
  compas converter : Subsystem
  xyz2GPS : PreScanUsefulBlocks/xyz2GPS  CoordinateCount=1  GPS_base=[0.000000 0.000000 0.000]
  x [m] : Outport
  y [m] : Outport  Port=2
  z [m] : Outport  Port=3
  rotx [deg] : Outport  Port=4
  roty [deg] : Outport  Port=5
  rotz [deg] : Outport  Port=6
  GPS lat [deg] : Outport  Port=7
  GPS long [deg] : Outport  Port=8
  GPS alt [m] : Outport  Port=9
  velocity [m/s] : Outport  Port=10
  heading [deg] : Outport  Port=11
  yaw rate [deg/s] : Outport  Port=12
  wires:
  Demux3/4 -> Gain1/1
  Gain1/1 -> yaw rate [deg/s]/1
  Demux3/3 -> velocity [m/s]/1
  compas converter/1(heading [deg]) -> heading [deg]/1
  xyz2GPS/1 -> Demux4/1
  Demux4/3 -> GPS alt [m]/1
  Demux4/2 -> GPS long [deg]/1
  Demux4/1 -> GPS lat [deg]/1
  Demux3/2 -> Gain/1, Selector/1
  Demux3/1 -> xyz2GPS/1, Demux1/1
  SELF/1 -> Demux3/1
  Demux2/3 -> rotz [deg]/1
  Demux2/2 -> roty [deg]/1
  Demux2/1 -> rotx [deg]/1
  Demux1/3 -> z [m]/1
  Demux1/2 -> y [m]/1
  Demux1/1 -> x [m]/1
  Gain/1 -> Demux2/1
  Selector/1 -> compas converter/1(rotz [rad])

== system ThreeDOF_cs/BMW_X5_1/Dynamics_Empty ==
  note: For state mode 'Dynamic' positions
      | are not taken into account, as they
      | are computed by integrating velocity.
      | Click annotation for Help.
  In1 : Inport
  Ground_{1..7} (7 alike) : Ground
  Integrator : Integrator
  MuxState : Subsystem  Tag=MuxState  mask(Empty Dynamics State Block){positioningmode=on, TimeStep=1/20}
      mask prompts: positioningmode "Positioning Mode"; TimeStep "Auto Assigned: Time Step [s]"
      mask help:
      | Build the state of an actor based on user input.
      | The user can either use positioning mode or dynamics mode.
      | - When using positioning mode the position and orientation of the actor are set directly based on the input. Expected input is relative to the initial position and orientation of the actor. It's also possible to specify the velocity of the actor, though this input isn't used, only passed on.
      | - When using dynamics mode the position input is ignored. Expected input is velocity and orientation. The velocity is relative the current orientation of the actor, while orientation is relative to its initial orientation. The position of the actor is calculated based on the velocity and orientation given.
      settings: DeleteFcn=PreScanBlockDeleteFcn;
  State : Outport  Tag=StateOutport
  wires:
  Integrator/1 -> MuxState/1(x [m])
  In1/1 -> MuxState/4(dx [m/s]), Integrator/1
  MuxState/1(state) -> State/1
  Ground_1/1 -> MuxState/2(y [m])
  Ground_2/1 -> MuxState/3(z [m])
  Ground_3/1 -> MuxState/5(dy [m/s])
  Ground_4/1 -> MuxState/6(dz [m/s])
  Ground_5/1 -> MuxState/7(R [rad])
  Ground_6/1 -> MuxState/8(P [rad])
  Ground_7/1 -> MuxState/9(Y [rad])

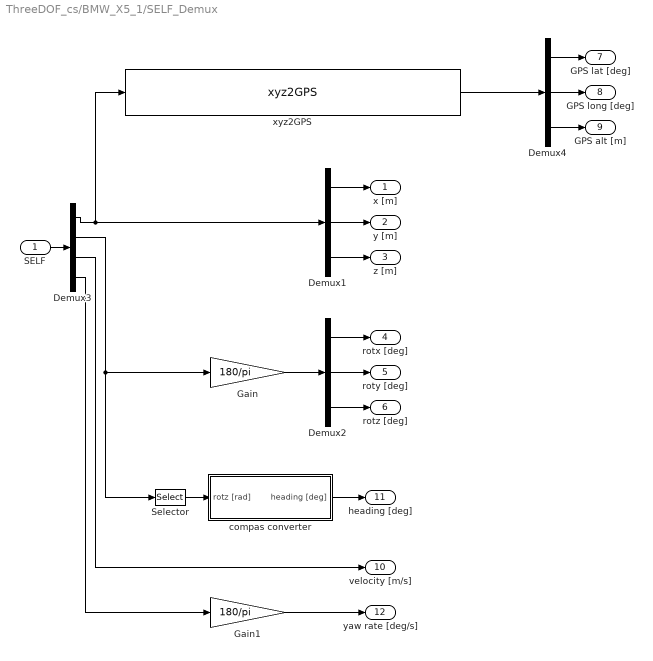
== system ThreeDOF_cs/BMW_X5_1/SELF_Demux ==
  SELF : Inport
  Demux1 : Demux  Outputs=3
  Demux2 : Demux  Outputs=3
  Demux3 : Demux  Outputs=[3 3 1 1]
  Demux4 : Demux  Outputs=3
  Gain : Gain  Gain=180/pi
  Gain1 : Gain  Gain=180/pi
  Selector : Selector  InputPortWidth=3  IndexOptions=Index vector (dialog)  Indices=[3]  OutputSizes=1
  compas converter : Subsystem
  xyz2GPS : PreScanUsefulBlocks/xyz2GPS  CoordinateCount=1  GPS_base=[0.000000 0.000000 0.000]
  x [m] : Outport
  y [m] : Outport  Port=2
  z [m] : Outport  Port=3
  rotx [deg] : Outport  Port=4
  roty [deg] : Outport  Port=5
  rotz [deg] : Outport  Port=6
  GPS lat [deg] : Outport  Port=7
  GPS long [deg] : Outport  Port=8
  GPS alt [m] : Outport  Port=9
  velocity [m/s] : Outport  Port=10
  heading [deg] : Outport  Port=11
  yaw rate [deg/s] : Outport  Port=12
  wires:
  Demux3/4 -> Gain1/1
  Gain1/1 -> yaw rate [deg/s]/1
  Demux3/3 -> velocity [m/s]/1
  compas converter/1(heading [deg]) -> heading [deg]/1
  xyz2GPS/1 -> Demux4/1
  Demux4/3 -> GPS alt [m]/1
  Demux4/2 -> GPS long [deg]/1
  Demux4/1 -> GPS lat [deg]/1
  Demux3/2 -> Gain/1, Selector/1
  Demux3/1 -> xyz2GPS/1, Demux1/1
  SELF/1 -> Demux3/1
  Demux2/3 -> rotz [deg]/1
  Demux2/2 -> roty [deg]/1
  Demux2/1 -> rotx [deg]/1
  Demux1/3 -> z [m]/1
  Demux1/2 -> y [m]/1
  Demux1/1 -> x [m]/1
  Gain/1 -> Demux2/1
  Selector/1 -> compas converter/1(rotz [rad])

== system ThreeDOF_cs/Fiat_Bravo_1/Dynamics_Empty ==
  note: For state mode 'Dynamic' positions
      | are not taken into account, as they
      | are computed by integrating velocity.
      | Click annotation for Help.
  In1 : Inport
  Ground_{1..7} (7 alike) : Ground
  Integrator : Integrator
  MuxState : Subsystem  Tag=MuxState  mask(Empty Dynamics State Block){positioningmode=on, TimeStep=1/20}
      mask prompts: positioningmode "Positioning Mode"; TimeStep "Auto Assigned: Time Step [s]"
      mask help:
      | Build the state of an actor based on user input.
      | The user can either use positioning mode or dynamics mode.
      | - When using positioning mode the position and orientation of the actor are set directly based on the input. Expected input is relative to the initial position and orientation of the actor. It's also possible to specify the velocity of the actor, though this input isn't used, only passed on.
      | - When using dynamics mode the position input is ignored. Expected input is velocity and orientation. The velocity is relative the current orientation of the actor, while orientation is relative to its initial orientation. The position of the actor is calculated based on the velocity and orientation given.
      settings: DeleteFcn=PreScanBlockDeleteFcn;
  State : Outport  Tag=StateOutport
  wires:
  Integrator/1 -> MuxState/1(x [m])
  In1/1 -> MuxState/4(dx [m/s]), Integrator/1
  MuxState/1(state) -> State/1
  Ground_1/1 -> MuxState/2(y [m])
  Ground_2/1 -> MuxState/3(z [m])
  Ground_3/1 -> MuxState/5(dy [m/s])
  Ground_4/1 -> MuxState/6(dz [m/s])
  Ground_5/1 -> MuxState/7(R [rad])
  Ground_6/1 -> MuxState/8(P [rad])
  Ground_7/1 -> MuxState/9(Y [rad])

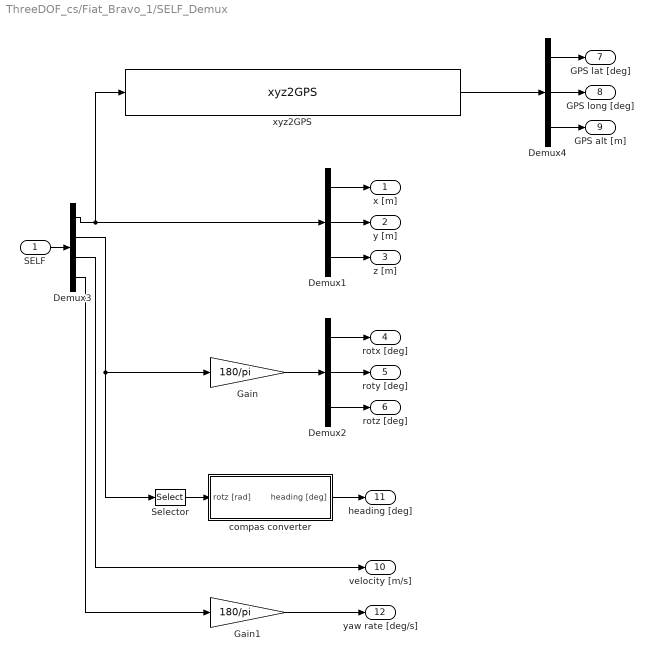
== system ThreeDOF_cs/Fiat_Bravo_1/SELF_Demux ==
  SELF : Inport
  Demux1 : Demux  Outputs=3
  Demux2 : Demux  Outputs=3
  Demux3 : Demux  Outputs=[3 3 1 1]
  Demux4 : Demux  Outputs=3
  Gain : Gain  Gain=180/pi
  Gain1 : Gain  Gain=180/pi
  Selector : Selector  InputPortWidth=3  IndexOptions=Index vector (dialog)  Indices=[3]  OutputSizes=1
  compas converter : Subsystem
  xyz2GPS : PreScanUsefulBlocks/xyz2GPS  CoordinateCount=1  GPS_base=[0.000000 0.000000 0.000]
  x [m] : Outport
  y [m] : Outport  Port=2
  z [m] : Outport  Port=3
  rotx [deg] : Outport  Port=4
  roty [deg] : Outport  Port=5
  rotz [deg] : Outport  Port=6
  GPS lat [deg] : Outport  Port=7
  GPS long [deg] : Outport  Port=8
  GPS alt [m] : Outport  Port=9
  velocity [m/s] : Outport  Port=10
  heading [deg] : Outport  Port=11
  yaw rate [deg/s] : Outport  Port=12
  wires:
  Demux3/4 -> Gain1/1
  Gain1/1 -> yaw rate [deg/s]/1
  Demux3/3 -> velocity [m/s]/1
  compas converter/1(heading [deg]) -> heading [deg]/1
  xyz2GPS/1 -> Demux4/1
  Demux4/3 -> GPS alt [m]/1
  Demux4/2 -> GPS long [deg]/1
  Demux4/1 -> GPS lat [deg]/1
  Demux3/2 -> Gain/1, Selector/1
  Demux3/1 -> xyz2GPS/1, Demux1/1
  SELF/1 -> Demux3/1
  Demux2/3 -> rotz [deg]/1
  Demux2/2 -> roty [deg]/1
  Demux2/1 -> rotx [deg]/1
  Demux1/3 -> z [m]/1
  Demux1/2 -> y [m]/1
  Demux1/1 -> x [m]/1
  Gain/1 -> Demux2/1
  Selector/1 -> compas converter/1(rotz [rad])

== system ThreeDOF_cs/STATE_Audi_A8_1/Acceleration ==
  Y : Inport
  Assignment : Assignment  IndexMode=Zero-based  SampleTime=TimeStep  IndexOptions=Starting index (dialog)  Indices=PortIndex  OutputSizes=[1 1]
  Data Store Read : DataStoreRead  DataStoreName=SimCoreActuators  SampleTime=TimeStep
  Data Store Write : DataStoreWrite  DataStoreName=SimCoreActuators
  wires:
  Assignment/1 -> Data Store Write/1
  Data Store Read/1 -> Assignment/1
  Y/1 -> Assignment/2

== system ThreeDOF_cs/STATE_Audi_A8_1/Position ==
  Y : Inport
  Assignment : Assignment  IndexMode=Zero-based  SampleTime=TimeStep  IndexOptions=Starting index (dialog)  Indices=PortIndex  OutputSizes=[1 1]
  Data Store Read : DataStoreRead  DataStoreName=SimCoreActuators  SampleTime=TimeStep
  Data Store Write : DataStoreWrite  DataStoreName=SimCoreActuators
  wires:
  Y/1 -> Assignment/2
  Data Store Read/1 -> Assignment/1
  Assignment/1 -> Data Store Write/1

== system ThreeDOF_cs/STATE_Audi_A8_1/RPY ==
  Y : Inport
  Assignment : Assignment  IndexMode=Zero-based  SampleTime=TimeStep  IndexOptions=Starting index (dialog)  Indices=PortIndex  OutputSizes=[1 1]
  Data Store Read : DataStoreRead  DataStoreName=SimCoreActuators  SampleTime=TimeStep
  Data Store Write : DataStoreWrite  DataStoreName=SimCoreActuators
  wires:
  Assignment/1 -> Data Store Write/1
  Data Store Read/1 -> Assignment/1
  Y/1 -> Assignment/2
